simulink model "Motor_model_with_Matlab_interface"  (R2019b)
settings: Solver=VariableStepAuto  StartTime=0.0  StopTime=180  RelTol=1e-3
settings Model: Creator=Олег  LastModifiedBy=Олег

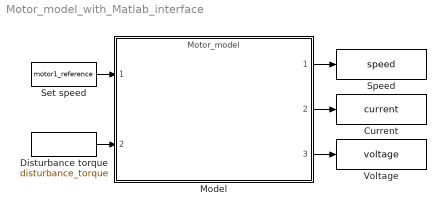
== system Motor_model_with_Matlab_interface ==
  Current : ToWorkspace  VariableName=current  SaveFormat=Timeseries  SampleTime=-1
  Disturbance torque : FromWorkspace  VariableName=disturbance_torque  SampleTime=0
  Model : ModelReference  ModelNameDialog=Motor_model.slx  SimulationMode=Normal  ModelReferenceVersion=1.143
  Set speed : FromWorkspace  VariableName=motor1_reference  SampleTime=0
  Speed : ToWorkspace  VariableName=speed  SaveFormat=Timeseries  SampleTime=-1
  Voltage : ToWorkspace  VariableName=voltage  SaveFormat=Timeseries  SampleTime=-1
  wires:
  Set speed/1 -> Model/1
  Disturbance torque/1 -> Model/2
  Model/1 -> Speed/1
  Model/2 -> Current/1
  Model/3 -> Voltage/1
